simulink model "gm_uz_JL_pmsmModel"  (R2025a)
settings: Solver=FixedStepDiscrete  StartTime=0.0  StopTime=1  RelTol=1e-3
libraries: hdlmdlgenlib x2
(part 2 of 2)

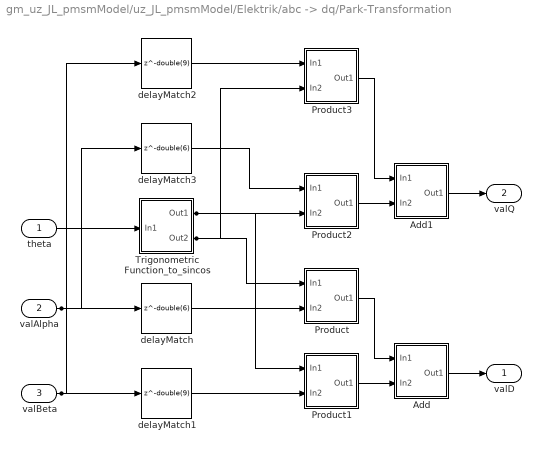
== system gm_uz_JL_pmsmModel/uz_JL_pmsmModel/Elektrik/abc -> dq/Park-Transformation ==
  theta : Inport  OutDataTypeStr=single  PortDimensions=1  SampleTime=2e-08
  valAlpha : Inport  Port=2  OutDataTypeStr=single  PortDimensions=1  SampleTime=2e-08
  valBeta : Inport  Port=3  OutDataTypeStr=single  PortDimensions=1  SampleTime=2e-08
  Add : Subsystem
      mask Display: disp('NFP\nadd');
  Add1 : Subsystem
      mask Display: disp('NFP\nadd');
  Product : Subsystem
      mask Display: disp('NFP\nmul');
  Product1 : Subsystem
      mask Display: disp('NFP\nmul');
  Product2 : Subsystem
      mask Display: disp('NFP\nmul');
  Product3 : Subsystem
      mask Display: disp('NFP\nmul');
  Trigonometric Function_to_sincos : Subsystem
      mask Display: disp('NFP\ntrig2');
  delayMatch : Delay  DelayLength=double(6)  InitialCondition=0  SampleTime=2e-08
  delayMatch1 : Delay  DelayLength=double(9)  InitialCondition=0  SampleTime=2e-08
  delayMatch2 : Delay  DelayLength=double(9)  InitialCondition=0  SampleTime=2e-08
  delayMatch3 : Delay  DelayLength=double(6)  InitialCondition=0  SampleTime=2e-08
  valD : Outport  SampleTime=2e-08
  valQ : Outport  Port=2  SampleTime=2e-08
  wires:
  Trigonometric Function_to_sincos/2(Out2) -> Product3/2(In2), Product/1(In1)
  theta/1 -> Trigonometric Function_to_sincos/1(In1)
  delayMatch2/1 -> Product3/1(In1)
  Trigonometric Function_to_sincos/1(Out1) -> Product1/1(In1), Product2/2(In2)
  delayMatch1/1 -> Product1/2(In2)
  valAlpha/1 -> delayMatch3/1, delayMatch/1
  Product2/1(Out1) -> Add1/2(In2)
  valBeta/1 -> delayMatch2/1, delayMatch1/1
  delayMatch3/1 -> Product2/1(In1)
  delayMatch/1 -> Product/2(In2)
  Product3/1(Out1) -> Add1/1(In1)
  Product/1(Out1) -> Add/1(In1)
  Product1/1(Out1) -> Add/2(In2)
  Add1/1(Out1) -> valQ/1
  Add/1(Out1) -> valD/1

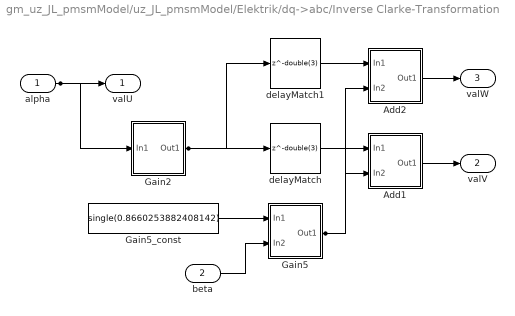
== system gm_uz_JL_pmsmModel/uz_JL_pmsmModel/Elektrik/dq->abc/Inverse Clarke-Transformation ==
  alpha : Inport  OutDataTypeStr=single  PortDimensions=1  SampleTime=2e-08
  beta : Inport  Port=2  OutDataTypeStr=single  PortDimensions=1  SampleTime=2e-08
  Add1 : Subsystem
      mask Display: disp('NFP\nadd');
  Add2 : Subsystem
      mask Display: disp('NFP\nadd');
  Gain2 : Subsystem
      mask Display: disp('NFP\ngain_pow2');
  Gain5 : Subsystem
      mask Display: disp('NFP\nmul');
  Gain5_const : Constant  Value=single(0.8660253882408142)  OutDataTypeStr=single  SampleTime=2e-08
  delayMatch : Delay  DelayLength=double(3)  InitialCondition=0  SampleTime=2e-08
  delayMatch1 : Delay  DelayLength=double(3)  InitialCondition=0  SampleTime=2e-08
  valU : Outport  SampleTime=2e-08
  valV : Outport  Port=2  SampleTime=2e-08
  valW : Outport  Port=3  SampleTime=2e-08
  wires:
  alpha/1 -> Gain2/1(In1), valU/1
  Gain2/1(Out1) -> delayMatch1/1, delayMatch/1
  Gain5_const/1 -> Gain5/1(In1)
  beta/1 -> Gain5/2(In2)
  Gain5/1(Out1) -> Add2/2(In2), Add1/2(In2)
  delayMatch1/1 -> Add2/1(In1)
  delayMatch/1 -> Add1/1(In1)
  Add2/1(Out1) -> valW/1
  Add1/1(Out1) -> valV/1

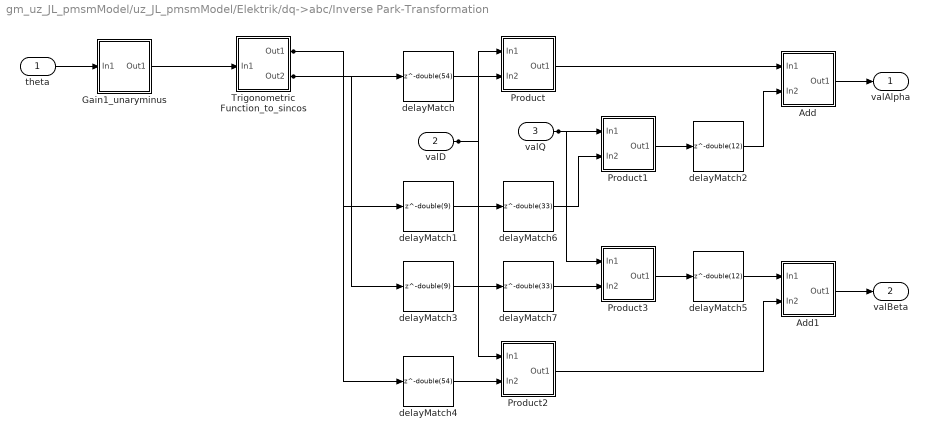
== system gm_uz_JL_pmsmModel/uz_JL_pmsmModel/Elektrik/dq->abc/Inverse Park-Transformation ==
  theta : Inport  OutDataTypeStr=single  PortDimensions=1  SampleTime=2e-08
  valD : Inport  Port=2  OutDataTypeStr=single  PortDimensions=1  SampleTime=2e-08
  valQ : Inport  Port=3  OutDataTypeStr=single  PortDimensions=1  SampleTime=2e-08
  Add : Subsystem
      mask Display: disp('NFP\nadd');
  Add1 : Subsystem
      mask Display: disp('NFP\nadd');
  Gain1_unaryminus : Subsystem
      mask Display: disp('NFP\numinus');
  Product : Subsystem
      mask Display: disp('NFP\nmul');
  Product1 : Subsystem
      mask Display: disp('NFP\nmul');
  Product2 : Subsystem
      mask Display: disp('NFP\nmul');
  Product3 : Subsystem
      mask Display: disp('NFP\nmul');
  Trigonometric Function_to_sincos : Subsystem
      mask Display: disp('NFP\ntrig2');
  delayMatch : Delay  DelayLength=double(54)  InitialCondition=0  SampleTime=2e-08
  delayMatch1 : Delay  DelayLength=double(9)  InitialCondition=0  SampleTime=2e-08
  delayMatch2 : Delay  DelayLength=double(12)  InitialCondition=0  SampleTime=2e-08
  delayMatch3 : Delay  DelayLength=double(9)  InitialCondition=0  SampleTime=2e-08
  delayMatch4 : Delay  DelayLength=double(54)  InitialCondition=0  SampleTime=2e-08
  delayMatch5 : Delay  DelayLength=double(12)  InitialCondition=0  SampleTime=2e-08
  delayMatch6 : Delay  DelayLength=double(33)  InitialCondition=0  SampleTime=2e-08
  delayMatch7 : Delay  DelayLength=double(33)  InitialCondition=0  SampleTime=2e-08
  valAlpha : Outport  SampleTime=2e-08
  valBeta : Outport  Port=2  SampleTime=2e-08
  wires:
  theta/1 -> Gain1_unaryminus/1(In1)
  delayMatch3/1 -> delayMatch7/1
  Gain1_unaryminus/1(Out1) -> Trigonometric Function_to_sincos/1(In1)
  delayMatch1/1 -> delayMatch6/1
  Trigonometric Function_to_sincos/1(Out1) -> delayMatch4/1, delayMatch1/1
  Trigonometric Function_to_sincos/2(Out2) -> delayMatch3/1, delayMatch/1
  valD/1 -> Product2/1(In1), Product/1(In1)
  delayMatch/1 -> Product/2(In2)
  delayMatch4/1 -> Product2/2(In2)
  Product/1(Out1) -> Add/1(In1)
  valQ/1 -> Product3/1(In1), Product1/1(In1)
  delayMatch6/1 -> Product1/2(In2)
  delayMatch7/1 -> Product3/2(In2)
  Product2/1(Out1) -> Add1/2(In2)
  Product1/1(Out1) -> delayMatch2/1
  Product3/1(Out1) -> delayMatch5/1
  delayMatch2/1 -> Add/2(In2)
  delayMatch5/1 -> Add1/1(In1)
  Add/1(Out1) -> valAlpha/1
  Add1/1(Out1) -> valBeta/1

== system gm_uz_JL_pmsmModel/uz_JL_pmsmModel/Mechanik/Drehmomentberechnung/Gain ==
  In1 : Inport
  In2 : Inport  Port=2
  Gain : Product  Inputs=**  OutDataTypeStr=single  SampleTime=2e-08
  Gain_pd1 : Delay  DelayLength=6
  Out1 : Outport
  wires:
  In1/1 -> Gain/1
  In2/1 -> Gain/2
  Gain/1 -> Gain_pd1/1
  Gain_pd1/1 -> Out1/1

== system gm_uz_JL_pmsmModel/uz_JL_pmsmModel/Mechanik/Drehmomentberechnung/Prduct_3 ==
  In1 : Inport
  In2 : Inport  Port=2
  Prduct_3 : Product  Inputs=**  OutDataTypeStr=single  SampleTime=2e-08
  Prduct_3_pd1 : Delay  DelayLength=6
  Out1 : Outport
  wires:
  In1/1 -> Prduct_3/1
  In2/1 -> Prduct_3/2
  Prduct_3/1 -> Prduct_3_pd1/1
  Prduct_3_pd1/1 -> Out1/1

== system gm_uz_JL_pmsmModel/uz_JL_pmsmModel/Mechanik/Drehmomentberechnung/Prduct_31 ==
  In1 : Inport
  In2 : Inport  Port=2
  Prduct_31 : Product  Inputs=**  OutDataTypeStr=single  SampleTime=2e-08
  Prduct_31_pd1 : Delay  DelayLength=6
  Out1 : Outport
  wires:
  In1/1 -> Prduct_31/1
  In2/1 -> Prduct_31/2
  Prduct_31/1 -> Prduct_31_pd1/1
  Prduct_31_pd1/1 -> Out1/1

== system gm_uz_JL_pmsmModel/uz_JL_pmsmModel/Mechanik/Drehmomentberechnung/Product1 ==
  In1 : Inport
  In2 : Inport  Port=2
  Product1 : Product  Inputs=**  OutDataTypeStr=single  SampleTime=2e-08
  Product1_pd1 : Delay  DelayLength=6
  Out1 : Outport
  wires:
  In1/1 -> Product1/1
  In2/1 -> Product1/2
  Product1/1 -> Product1_pd1/1
  Product1_pd1/1 -> Out1/1

== system gm_uz_JL_pmsmModel/uz_JL_pmsmModel/Mechanik/Drehmomentberechnung/Product2 ==
  In1 : Inport
  In2 : Inport  Port=2
  Product2 : Product  Inputs=**  OutDataTypeStr=single  SampleTime=2e-08
  Product2_pd1 : Delay  DelayLength=6
  Out1 : Outport
  wires:
  In1/1 -> Product2/1
  In2/1 -> Product2/2
  Product2/1 -> Product2_pd1/1
  Product2_pd1/1 -> Out1/1

== system gm_uz_JL_pmsmModel/uz_JL_pmsmModel/Mechanik/Drehmomentberechnung/Subtract ==
  In1 : Inport
  In2 : Inport  Port=2
  Subtract : Sum  Inputs=+-  OutDataTypeStr=single  SampleTime=2e-08
  Subtract_pd1 : Delay  DelayLength=6
  Out1 : Outport
  wires:
  In1/1 -> Subtract/1
  In2/1 -> Subtract/2
  Subtract/1 -> Subtract_pd1/1
  Subtract_pd1/1 -> Out1/1

== system gm_uz_JL_pmsmModel/uz_JL_pmsmModel/Mechanik/Drehmomentberechnung/Subtract1 ==
  In1 : Inport
  In2 : Inport  Port=2
  Subtract1 : Sum  OutDataTypeStr=single  SampleTime=2e-08
  Subtract1_pd1 : Delay  DelayLength=6
  Out1 : Outport
  wires:
  In1/1 -> Subtract1/1
  In2/1 -> Subtract1/2
  Subtract1/1 -> Subtract1_pd1/1
  Subtract1_pd1/1 -> Out1/1

== system gm_uz_JL_pmsmModel/uz_JL_pmsmModel/Mechanik/Subsystem1/Abs ==
  In1 : Inport
  Abs : Abs  SampleTime=2e-08  OutDataTypeStr=single  RndMeth=Nearest  SaturateOnIntegerOverflow=off
  Out1 : Outport
  wires:
  In1/1 -> Abs/1
  Abs/1 -> Out1/1

== system gm_uz_JL_pmsmModel/uz_JL_pmsmModel/Mechanik/Subsystem1/Add ==
  In1 : Inport
  In2 : Inport  Port=2
  Add : Sum  OutDataTypeStr=single  SampleTime=2e-08
  Add_pd1 : Delay  DelayLength=6
  Out1 : Outport
  wires:
  In1/1 -> Add/1
  In2/1 -> Add/2
  Add/1 -> Add_pd1/1
  Add_pd1/1 -> Out1/1

== system gm_uz_JL_pmsmModel/uz_JL_pmsmModel/Mechanik/Subsystem1/Add1 ==
  In1 : Inport
  In2 : Inport  Port=2
  Add1 : Sum  OutDataTypeStr=single  SampleTime=2e-08
  Add1_pd1 : Delay  DelayLength=6
  Out1 : Outport
  wires:
  In1/1 -> Add1/1
  In2/1 -> Add1/2
  Add1/1 -> Add1_pd1/1
  Add1_pd1/1 -> Out1/1

== system gm_uz_JL_pmsmModel/uz_JL_pmsmModel/Mechanik/Subsystem1/Compare To Constant1_relop ==
  In1 : Inport
  In2 : Inport  Port=2
  Compare To Constant1_relop : RelationalOperator  OutDataTypeStr=boolean  SampleTime=2e-08
  Compare To Constant1_relop_pd1 : Delay  DelayLength=1
  Out1 : Outport
  wires:
  In1/1 -> Compare To Constant1_relop/1
  In2/1 -> Compare To Constant1_relop/2
  Compare To Constant1_relop/1 -> Compare To Constant1_relop_pd1/1
  Compare To Constant1_relop_pd1/1 -> Out1/1

== system gm_uz_JL_pmsmModel/uz_JL_pmsmModel/Mechanik/Subsystem1/Product ==
  In1 : Inport
  In2 : Inport  Port=2
  Product : Product  Inputs=**  OutDataTypeStr=single  SampleTime=2e-08
  Product_pd1 : Delay  DelayLength=6
  Out1 : Outport
  wires:
  In1/1 -> Product/1
  In2/1 -> Product/2
  Product/1 -> Product_pd1/1
  Product_pd1/1 -> Out1/1

== system gm_uz_JL_pmsmModel/uz_JL_pmsmModel/Mechanik/Subsystem1/Product1 ==
  In1 : Inport
  In2 : Inport  Port=2
  Product1 : Product  Inputs=**  OutDataTypeStr=single  SampleTime=2e-08
  Product1_pd1 : Delay  DelayLength=6
  Out1 : Outport
  wires:
  In1/1 -> Product1/1
  In2/1 -> Product1/2
  Product1/1 -> Product1_pd1/1
  Product1_pd1/1 -> Out1/1

== system gm_uz_JL_pmsmModel/uz_JL_pmsmModel/Mechanik/Subsystem1/Product2 ==
  In1 : Inport
  In2 : Inport  Port=2
  Product2 : Product  Inputs=**  OutDataTypeStr=single  SampleTime=2e-08
  Product2_pd1 : Delay  DelayLength=6
  Out1 : Outport
  wires:
  In1/1 -> Product2/1
  In2/1 -> Product2/2
  Product2/1 -> Product2_pd1/1
  Product2_pd1/1 -> Out1/1

== system gm_uz_JL_pmsmModel/uz_JL_pmsmModel/Mechanik/Subsystem1/Product3 ==
  In1 : Inport
  In2 : Inport  Port=2
  Product3 : Product  Inputs=**  OutDataTypeStr=single  SampleTime=2e-08
  Product3_pd1 : Delay  DelayLength=6
  Out1 : Outport
  wires:
  In1/1 -> Product3/1
  In2/1 -> Product3/2
  Product3/1 -> Product3_pd1/1
  Product3_pd1/1 -> Out1/1

== system gm_uz_JL_pmsmModel/uz_JL_pmsmModel/Mechanik/Subsystem1/Product4 ==
  In1 : Inport
  In2 : Inport  Port=2
  Product4 : Product  Inputs=**  OutDataTypeStr=single  SampleTime=2e-08
  Product4_pd1 : Delay  DelayLength=6
  Out1 : Outport
  wires:
  In1/1 -> Product4/1
  In2/1 -> Product4/2
  Product4/1 -> Product4_pd1/1
  Product4_pd1/1 -> Out1/1

== system gm_uz_JL_pmsmModel/uz_JL_pmsmModel/Mechanik/Subsystem1/Sign ==
  In1 : Inport
  Sign : Signum  SampleTime=2e-08
  Out1 : Outport
  wires:
  In1/1 -> Sign/1
  Sign/1 -> Out1/1

== system gm_uz_JL_pmsmModel/uz_JL_pmsmModel/Mechanik/Subsystem1/Subtract ==
  In1 : Inport
  In2 : Inport  Port=2
  Subtract : Sum  Inputs=+-  OutDataTypeStr=single  SampleTime=2e-08
  Subtract_pd1 : Delay  DelayLength=6
  Out1 : Outport
  wires:
  In1/1 -> Subtract/1
  In2/1 -> Subtract/2
  Subtract/1 -> Subtract_pd1/1
  Subtract_pd1/1 -> Out1/1

== system gm_uz_JL_pmsmModel/uz_JL_pmsmModel/Mechanik/Subsystem1/adder ==
  In1 : Inport
  In2 : Inport  Port=2
  adder : Sum  OutDataTypeStr=single  RndMeth=Simplest  SampleTime=2e-08
  adder_pd1 : Delay  DelayLength=6
  Out1 : Outport
  wires:
  In1/1 -> adder/1
  In2/1 -> adder/2
  adder/1 -> adder_pd1/1
  adder_pd1/1 -> Out1/1

== system gm_uz_JL_pmsmModel/uz_JL_pmsmModel/Mechanik/Subsystem1/adder1 ==
  In1 : Inport
  In2 : Inport  Port=2
  adder1 : Sum  OutDataTypeStr=single  RndMeth=Simplest  SampleTime=2e-08
  adder1_pd1 : Delay  DelayLength=6
  Out1 : Outport
  wires:
  In1/1 -> adder1/1
  In2/1 -> adder1/2
  adder1/1 -> adder1_pd1/1
  adder1_pd1/1 -> Out1/1

== system gm_uz_JL_pmsmModel/uz_JL_pmsmModel/Mechanik/Subsystem1/gain ==
  In1 : Inport
  In2 : Inport  Port=2
  gain : Product  Inputs=**  OutDataTypeStr=single  RndMeth=Simplest  SampleTime=2e-08
  gain_pd1 : Delay  DelayLength=6
  Out1 : Outport
  wires:
  In1/1 -> gain/1
  In2/1 -> gain/2
  gain/1 -> gain_pd1/1
  gain_pd1/1 -> Out1/1

== system gm_uz_JL_pmsmModel/uz_JL_pmsmModel/Elektrik/abc -> dq/Clark Transformation/Add1 ==
  In1 : Inport
  In2 : Inport  Port=2
  Add1 : Sum  OutDataTypeStr=single  SampleTime=2e-08
  Add1_pd1 : Delay  DelayLength=6
  Out1 : Outport
  wires:
  In1/1 -> Add1/1
  In2/1 -> Add1/2
  Add1/1 -> Add1_pd1/1
  Add1_pd1/1 -> Out1/1

== system gm_uz_JL_pmsmModel/uz_JL_pmsmModel/Elektrik/abc -> dq/Clark Transformation/Add_stage2 ==
  In1 : Inport
  In2 : Inport  Port=2
  Add_stage2 : Sum  OutDataTypeStr=single  SampleTime=2e-08
  Add_stage2_pd1 : Delay  DelayLength=6
  Out1 : Outport
  wires:
  In1/1 -> Add_stage2/1
  In2/1 -> Add_stage2/2
  Add_stage2/1 -> Add_stage2_pd1/1
  Add_stage2_pd1/1 -> Out1/1

== system gm_uz_JL_pmsmModel/uz_JL_pmsmModel/Elektrik/abc -> dq/Clark Transformation/Add_stage3 ==
  In1 : Inport
  In2 : Inport  Port=2
  Add_stage3 : Sum  OutDataTypeStr=single  SampleTime=2e-08
  Add_stage3_pd1 : Delay  DelayLength=6
  Out1 : Outport
  wires:
  In1/1 -> Add_stage3/1
  In2/1 -> Add_stage3/2
  Add_stage3/1 -> Add_stage3_pd1/1
  Add_stage3_pd1/1 -> Out1/1

== system gm_uz_JL_pmsmModel/uz_JL_pmsmModel/Elektrik/abc -> dq/Clark Transformation/Gain ==
  In1 : Inport
  In2 : Inport  Port=2
  Gain : Product  Inputs=**  OutDataTypeStr=single  SampleTime=2e-08
  Gain_pd1 : Delay  DelayLength=6
  Out1 : Outport
  wires:
  In1/1 -> Gain/1
  In2/1 -> Gain/2
  Gain/1 -> Gain_pd1/1
  Gain_pd1/1 -> Out1/1

== system gm_uz_JL_pmsmModel/uz_JL_pmsmModel/Elektrik/abc -> dq/Clark Transformation/Gain1 ==
  In1 : Inport
  In2 : Inport  Port=2
  Gain1 : Product  Inputs=**  OutDataTypeStr=single  SampleTime=2e-08
  Gain1_pd1 : Delay  DelayLength=6
  Out1 : Outport
  wires:
  In1/1 -> Gain1/1
  In2/1 -> Gain1/2
  Gain1/1 -> Gain1_pd1/1
  Gain1_pd1/1 -> Out1/1

== system gm_uz_JL_pmsmModel/uz_JL_pmsmModel/Elektrik/abc -> dq/Clark Transformation/Gain2 ==
  In1 : Inport
  Gain2 : Gain  Gain=single(-0.5)
  Gain2_pd1 : Delay  DelayLength=3
  Out1 : Outport
  wires:
  In1/1 -> Gain2/1
  Gain2/1 -> Gain2_pd1/1
  Gain2_pd1/1 -> Out1/1

== system gm_uz_JL_pmsmModel/uz_JL_pmsmModel/Elektrik/abc -> dq/Clark Transformation/Gain5 ==
  In1 : Inport
  In2 : Inport  Port=2
  Gain5 : Product  Inputs=**  OutDataTypeStr=single  SampleTime=2e-08
  Gain5_pd1 : Delay  DelayLength=6
  Out1 : Outport
  wires:
  In1/1 -> Gain5/1
  In2/1 -> Gain5/2
  Gain5/1 -> Gain5_pd1/1
  Gain5_pd1/1 -> Out1/1

== system gm_uz_JL_pmsmModel/uz_JL_pmsmModel/Elektrik/abc -> dq/Clark Transformation/Gain7 ==
  In1 : Inport
  Gain7 : Gain  Gain=single(-0.5)
  Gain7_pd1 : Delay  DelayLength=3
  Out1 : Outport
  wires:
  In1/1 -> Gain7/1
  Gain7/1 -> Gain7_pd1/1
  Gain7_pd1/1 -> Out1/1

== system gm_uz_JL_pmsmModel/uz_JL_pmsmModel/Elektrik/abc -> dq/Clark Transformation/sqrt(3)//2 ==
  In1 : Inport
  In2 : Inport  Port=2
  sqrt(3)/2 : Product  Inputs=**  OutDataTypeStr=single  SampleTime=2e-08
  sqrt(3)/2_pd1 : Delay  DelayLength=6
  Out1 : Outport
  wires:
  In1/1 -> sqrt(3)/2/1
  In2/1 -> sqrt(3)/2/2
  sqrt(3)/2/1 -> sqrt(3)/2_pd1/1
  sqrt(3)/2_pd1/1 -> Out1/1

== system gm_uz_JL_pmsmModel/uz_JL_pmsmModel/Elektrik/abc -> dq/Park-Transformation/Add ==
  In1 : Inport
  In2 : Inport  Port=2
  Add : Sum  OutDataTypeStr=single  SampleTime=2e-08
  Add_pd1 : Delay  DelayLength=6
  Out1 : Outport
  wires:
  In1/1 -> Add/1
  In2/1 -> Add/2
  Add/1 -> Add_pd1/1
  Add_pd1/1 -> Out1/1

== system gm_uz_JL_pmsmModel/uz_JL_pmsmModel/Elektrik/abc -> dq/Park-Transformation/Add1 ==
  In1 : Inport
  In2 : Inport  Port=2
  Add1 : Sum  Inputs=+-  OutDataTypeStr=single  SampleTime=2e-08
  Add1_pd1 : Delay  DelayLength=6
  Out1 : Outport
  wires:
  In1/1 -> Add1/1
  In2/1 -> Add1/2
  Add1/1 -> Add1_pd1/1
  Add1_pd1/1 -> Out1/1

== system gm_uz_JL_pmsmModel/uz_JL_pmsmModel/Elektrik/abc -> dq/Park-Transformation/Product ==
  In1 : Inport
  In2 : Inport  Port=2
  Product : Product  Inputs=**  OutDataTypeStr=single  SampleTime=2e-08
  Product_pd1 : Delay  DelayLength=6
  Out1 : Outport
  wires:
  In1/1 -> Product/1
  In2/1 -> Product/2
  Product/1 -> Product_pd1/1
  Product_pd1/1 -> Out1/1

== system gm_uz_JL_pmsmModel/uz_JL_pmsmModel/Elektrik/abc -> dq/Park-Transformation/Product1 ==
  In1 : Inport
  In2 : Inport  Port=2
  Product1 : Product  Inputs=**  OutDataTypeStr=single  SampleTime=2e-08
  Product1_pd1 : Delay  DelayLength=6
  Out1 : Outport
  wires:
  In1/1 -> Product1/1
  In2/1 -> Product1/2
  Product1/1 -> Product1_pd1/1
  Product1_pd1/1 -> Out1/1

== system gm_uz_JL_pmsmModel/uz_JL_pmsmModel/Elektrik/abc -> dq/Park-Transformation/Product2 ==
  In1 : Inport
  In2 : Inport  Port=2
  Product2 : Product  Inputs=**  OutDataTypeStr=single  SampleTime=2e-08
  Product2_pd1 : Delay  DelayLength=6
  Out1 : Outport
  wires:
  In1/1 -> Product2/1
  In2/1 -> Product2/2
  Product2/1 -> Product2_pd1/1
  Product2_pd1/1 -> Out1/1

== system gm_uz_JL_pmsmModel/uz_JL_pmsmModel/Elektrik/abc -> dq/Park-Transformation/Product3 ==
  In1 : Inport
  In2 : Inport  Port=2
  Product3 : Product  Inputs=**  OutDataTypeStr=single  SampleTime=2e-08
  Product3_pd1 : Delay  DelayLength=6
  Out1 : Outport
  wires:
  In1/1 -> Product3/1
  In2/1 -> Product3/2
  Product3/1 -> Product3_pd1/1
  Product3_pd1/1 -> Out1/1

== system gm_uz_JL_pmsmModel/uz_JL_pmsmModel/Elektrik/abc -> dq/Park-Transformation/Trigonometric Function_to_sincos ==
  In1 : Inport
  Trigonometric Function_to_sincos : Trigonometry  Operator=sincos  SampleTime=2e-08
  Trigonometric Function_to_sincos_pd1 : Delay  DelayLength=27
  Trigonometric Function_to_sincos_pd2 : Delay  DelayLength=27
  Out1 : Outport
  Out2 : Outport  Port=2
  wires:
  In1/1 -> Trigonometric Function_to_sincos/1
  Trigonometric Function_to_sincos/1 -> Trigonometric Function_to_sincos_pd1/1
  Trigonometric Function_to_sincos_pd1/1 -> Out1/1
  Trigonometric Function_to_sincos/2 -> Trigonometric Function_to_sincos_pd2/1
  Trigonometric Function_to_sincos_pd2/1 -> Out2/1

== system gm_uz_JL_pmsmModel/uz_JL_pmsmModel/Elektrik/dq->abc/Inverse Clarke-Transformation/Add1 ==
  In1 : Inport
  In2 : Inport  Port=2
  Add1 : Sum  OutDataTypeStr=single  SampleTime=2e-08
  Add1_pd1 : Delay  DelayLength=6
  Out1 : Outport
  wires:
  In1/1 -> Add1/1
  In2/1 -> Add1/2
  Add1/1 -> Add1_pd1/1
  Add1_pd1/1 -> Out1/1

== system gm_uz_JL_pmsmModel/uz_JL_pmsmModel/Elektrik/dq->abc/Inverse Clarke-Transformation/Add2 ==
  In1 : Inport
  In2 : Inport  Port=2
  Add2 : Sum  Inputs=+-  OutDataTypeStr=single  SampleTime=2e-08
  Add2_pd1 : Delay  DelayLength=6
  Out1 : Outport
  wires:
  In1/1 -> Add2/1
  In2/1 -> Add2/2
  Add2/1 -> Add2_pd1/1
  Add2_pd1/1 -> Out1/1

== system gm_uz_JL_pmsmModel/uz_JL_pmsmModel/Elektrik/dq->abc/Inverse Clarke-Transformation/Gain2 ==
  In1 : Inport
  Gain2 : Gain  Gain=single(-0.5)
  Gain2_pd1 : Delay  DelayLength=3
  Out1 : Outport
  wires:
  In1/1 -> Gain2/1
  Gain2/1 -> Gain2_pd1/1
  Gain2_pd1/1 -> Out1/1

== system gm_uz_JL_pmsmModel/uz_JL_pmsmModel/Elektrik/dq->abc/Inverse Clarke-Transformation/Gain5 ==
  In1 : Inport
  In2 : Inport  Port=2
  Gain5 : Product  Inputs=**  OutDataTypeStr=single  SampleTime=2e-08
  Gain5_pd1 : Delay  DelayLength=6
  Out1 : Outport
  wires:
  In1/1 -> Gain5/1
  In2/1 -> Gain5/2
  Gain5/1 -> Gain5_pd1/1
  Gain5_pd1/1 -> Out1/1

== system gm_uz_JL_pmsmModel/uz_JL_pmsmModel/Elektrik/dq->abc/Inverse Park-Transformation/Add ==
  In1 : Inport
  In2 : Inport  Port=2
  Add : Sum  OutDataTypeStr=single  SampleTime=2e-08
  Add_pd1 : Delay  DelayLength=6
  Out1 : Outport
  wires:
  In1/1 -> Add/1
  In2/1 -> Add/2
  Add/1 -> Add_pd1/1
  Add_pd1/1 -> Out1/1

== system gm_uz_JL_pmsmModel/uz_JL_pmsmModel/Elektrik/dq->abc/Inverse Park-Transformation/Add1 ==
  In1 : Inport
  In2 : Inport  Port=2
  Add1 : Sum  Inputs=+-  OutDataTypeStr=single  SampleTime=2e-08
  Add1_pd1 : Delay  DelayLength=6
  Out1 : Outport
  wires:
  In1/1 -> Add1/1
  In2/1 -> Add1/2
  Add1/1 -> Add1_pd1/1
  Add1_pd1/1 -> Out1/1

== system gm_uz_JL_pmsmModel/uz_JL_pmsmModel/Elektrik/dq->abc/Inverse Park-Transformation/Gain1_unaryminus ==
  In1 : Inport
  Gain1_unaryminus : UnaryMinus  SampleTime=2e-08
  Out1 : Outport
  wires:
  In1/1 -> Gain1_unaryminus/1
  Gain1_unaryminus/1 -> Out1/1

== system gm_uz_JL_pmsmModel/uz_JL_pmsmModel/Elektrik/dq->abc/Inverse Park-Transformation/Product ==
  In1 : Inport
  In2 : Inport  Port=2
  Product : Product  Inputs=**  OutDataTypeStr=single  SampleTime=2e-08
  Product_pd1 : Delay  DelayLength=6
  Out1 : Outport
  wires:
  In1/1 -> Product/1
  In2/1 -> Product/2
  Product/1 -> Product_pd1/1
  Product_pd1/1 -> Out1/1

== system gm_uz_JL_pmsmModel/uz_JL_pmsmModel/Elektrik/dq->abc/Inverse Park-Transformation/Product1 ==
  In1 : Inport
  In2 : Inport  Port=2
  Product1 : Product  Inputs=**  OutDataTypeStr=single  SampleTime=2e-08
  Product1_pd1 : Delay  DelayLength=6
  Out1 : Outport
  wires:
  In1/1 -> Product1/1
  In2/1 -> Product1/2
  Product1/1 -> Product1_pd1/1
  Product1_pd1/1 -> Out1/1

== system gm_uz_JL_pmsmModel/uz_JL_pmsmModel/Elektrik/dq->abc/Inverse Park-Transformation/Product2 ==
  In1 : Inport
  In2 : Inport  Port=2
  Product2 : Product  Inputs=**  OutDataTypeStr=single  SampleTime=2e-08
  Product2_pd1 : Delay  DelayLength=6
  Out1 : Outport
  wires:
  In1/1 -> Product2/1
  In2/1 -> Product2/2
  Product2/1 -> Product2_pd1/1
  Product2_pd1/1 -> Out1/1

== system gm_uz_JL_pmsmModel/uz_JL_pmsmModel/Elektrik/dq->abc/Inverse Park-Transformation/Product3 ==
  In1 : Inport
  In2 : Inport  Port=2
  Product3 : Product  Inputs=**  OutDataTypeStr=single  SampleTime=2e-08
  Product3_pd1 : Delay  DelayLength=6
  Out1 : Outport
  wires:
  In1/1 -> Product3/1
  In2/1 -> Product3/2
  Product3/1 -> Product3_pd1/1
  Product3_pd1/1 -> Out1/1

== system gm_uz_JL_pmsmModel/uz_JL_pmsmModel/Elektrik/dq->abc/Inverse Park-Transformation/Trigonometric Function_to_sincos ==
  In1 : Inport
  Trigonometric Function_to_sincos : Trigonometry  Operator=sincos  SampleTime=2e-08
  Trigonometric Function_to_sincos_pd1 : Delay  DelayLength=27
  Trigonometric Function_to_sincos_pd2 : Delay  DelayLength=27
  Out1 : Outport
  Out2 : Outport  Port=2
  wires:
  In1/1 -> Trigonometric Function_to_sincos/1
  Trigonometric Function_to_sincos/1 -> Trigonometric Function_to_sincos_pd1/1
  Trigonometric Function_to_sincos_pd1/1 -> Out1/1
  Trigonometric Function_to_sincos/2 -> Trigonometric Function_to_sincos_pd2/1
  Trigonometric Function_to_sincos_pd2/1 -> Out2/1
